simulink library "ZumoBotLib"  (R2014a)
settings: Solver=ode45  StartTime=0.0  StopTime=10.0  RelTol=1e-3
libraries: simulink x4, arduinolib x4
settings Model: Creator=cgupta  LastModifiedBy=cgupta

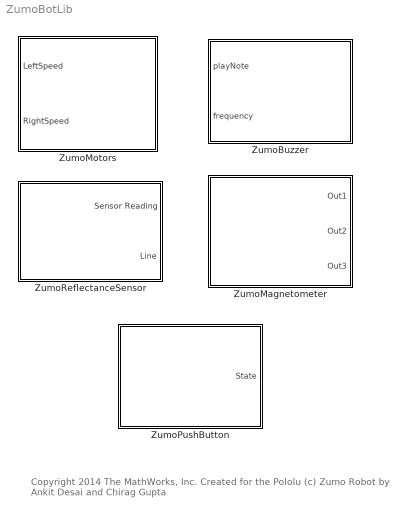
== system ZumoBotLib ==
  note: Copyright 2014 The MathWorks, Inc.
      | Created for the Pololu (c)  Zumo Robot by Ankit Desai and Chirag Gupta
  ZumoBuzzer : Subsystem  mask(Zumo Buzzer){}
      mask help:
      | This block provides access to the piezo buzzer on the ZumoBot.
      | The Block takes 2 inputs:
      | Enable: That enables the Buzzer
      | Frequency: That plays the specified frequency on the buzzer.
      mask Help:
      | This block provides access to the piezo buzzer on the ZumoBot.
      | The Block takes 2 inputs:
      | Enable: That enables the Buzzer
      | Frequency: That plays the specified frequency on the buzzer.
      mask Display:
      | image('zumobuzzer.jpg')
      | port_label('input',1,'Enable')
      | port_label('input',2,'Frequency')
  ZumoMagnetometer : Subsystem  mask(Zumo LSM303 Block){sampletime_lsm=0.2, debug_lsm=off, minX_lsm=-2048, maxX_lsm=2048, minY_lsm=-2048, maxY_lsm=2048, minZ_lsm=-4096, maxZ_lsm=4096}
      mask prompts: sampletime_lsm "Sample Time"; debug_lsm "Debug"; minX_lsm "Min Compass X"; maxX_lsm "Max Compass X"; minY_lsm "Min Compass Y"; maxY_lsm "Max Compass Y"; minZ_lsm "Min Compass Z"; maxZ_lsm "Max Compass Z"
      mask help:
      | This block provides acceleration as well as compass values.
      |
      | The output ports are: Acceleration and Compass respectively.
      |
      | The individual X, Y and Z values can be accessed from the bus for each.
      |
      | The SampleTime Parameter should be greater that 0.01.
      | The Debug checkbox enables debug Serial Print.
      |
      | The Min/Max Compass Readings can be calibrated to get accurate readings from the Magnetometer.
      mask Help:
      | This block provides acceleration as well as compass values.
      | 
      | The output ports are: Acceleration and Compass respectively.
      | 
      | The individual X, Y and Z values can be accessed from the bus for each.
      | 
      | The SampleTime Parameter should be greater that 0.01.
      | The Debug checkbox enables debug Serial Print.
      mask Display:
      | image('LSM_Magnetometer.jpg');
      | port_label('output',1,'Acceleration');
      | port_label('output',2,'Compass');
      | port_label('output',3,'Heading');
  ZumoMotors : Subsystem  mask(Zumo Motors){flipLeft=off, flipRight=off}
      mask prompts: flipLeft "Flip Left Motors"; flipRight "Flip Right Motors"
      mask help:
      | This Block allows you to control the speed and direction of the motors of
      | the ZumoBot.
      |
      | The ZumoMotors block accepts speed in the range of -255 to 255 where the
      | negative sign reverse direction of the motor.
      |
      | Incase one of your motors is configured to the contrary (- denotes forward
      | motion), you can set the flipLeft(/Right) motor flag on the block to
      | correct this.
      mask Display:
      | image('ZumoMotors.jpg')
      | port_label('input',1,'LeftSpeed')
      | port_label('input',2,'RightSpeed')
  ZumoPushButton : Subsystem  mask(Zumo Push Button){sampleTime_push=0.2}
      mask prompts: sampleTime_push "Sample Time"
      mask help:
      | This block provides access to the Push Button on the ZumoBot.
      |
      | The State returned is HIGH when the button is pressed, else LOW.
      mask Help:
      | This block provides access to the Push Button on the ZumoBot.
      | 
      | The State returned is HIGH when the button is pressed, else LOW.
      mask Display:
      | image('Zumo_push.jpg');
      | port_label('output',1,'State');
  ZumoReflectanceSensor : Subsystem  mask(Zumo Reflectance Sensor){sampleTime_dd=0.1, emitterPin_dd=255, debug_dd=off}
      mask prompts: sampleTime_dd "Sample Time"; emitterPin_dd "Emitter Pin"; debug_dd "Debug"
      mask help:
      | This is the driver block to access the Reflectance Sensor on the Zumo bot.
      | This block returns the raw sensor values of the each individual sensor as
      | well as the averaged line indicator.
      |
      | The Line Indicator has a value range from 0 - 5000 where 0 represents that
      | the line is underneath sensor 0 and 5000 represents that the line is under
      | sensor 6.
      | The Raw values of each sensor range from 0 - 2000.
      | The SampleTime Parameter should be greater that 0.01.
      | The Debug Checkbox enables debug Serial Print.
      |
      | The Emitter Pin is diasbled at 255, which signifies that the sensor
      | emitters are always on.
      mask TypeOptions emitterPin_dd: 255 | 1 | 0
      mask Display:
      | image('ZumoReflectanceArray.jpg',[0,0,0.75,1]);
      | port_label('output',1,'RawValues');
      | port_label('output',2,'Line');

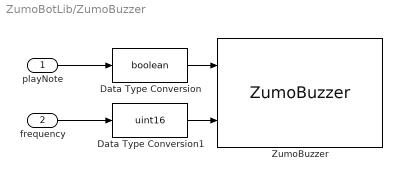
== system ZumoBotLib/ZumoBuzzer ==
  playNote : Inport
  frequency : Inport  Port=2
  Data Type Conversion : DataTypeConversion  OutDataTypeStr=boolean
  Data Type Conversion1 : DataTypeConversion  OutDataTypeStr=uint16
  ZumoBuzzer : S-Function  InitFcn=try, set_param(gcb,'FunctionName','ZumoBuzzer'), end  FunctionName=ZumoBuzzer  SFunctionModules=ZumoBuzzer_wrapper  EnableBusSupport=off  mask(S-Function Builder){frequency_zumobuzzer=0}
      mask prompts: frequency_zumobuzzer "Frequency"
      mask help: Simulink:masks:SFunctionBuilder_MD
      mask init:
      | val = [[.9  0.75 0.75 1 1 .9 .9 1]',[1 1 0.75 0.75 .9 .9 1 .9]'];try , sys = get_param(gcb,'SfunBuilderFcnName');if isempty(sys), sys = get_param(gcb,'FunctionName'); end,catch, sys = get_param(gcb,'FunctionName'); end
      settings: PreSaveFcn=try, set_param(gcb,'FunctionName','ZumoBuzzer'), end  OpenFcn=sfunctionwizard(gcbh)
      mask Display: plot(val(:,1),val(:,2)),disp(sys), port_label('input',1,'playTone'), port_label('input',2,'frequency')
  wires:
  playNote/1 -> Data Type Conversion/1
  Data Type Conversion/1 -> ZumoBuzzer/1
  Data Type Conversion1/1 -> ZumoBuzzer/2
  frequency/1 -> Data Type Conversion1/1

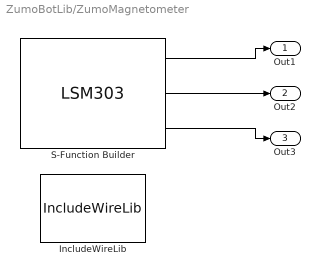
== system ZumoBotLib/ZumoMagnetometer ==
  IncludeWireLib : S-Function  InitFcn=try, set_param(gcb,'FunctionName','IncludeWireLib'), end  FunctionName=IncludeWireLib  SFunctionModules=IncludeWireLib_wrapper  EnableBusSupport=off  mask(S-Function Builder){}
      mask help: Simulink:masks:SFunctionBuilder_MD
      mask init: same as ZumoBotLib/ZumoBuzzer/ZumoBuzzer
      settings: PreSaveFcn=try, set_param(gcb,'FunctionName','IncludeWireLib'), end  OpenFcn=sfunctionwizard(gcbh)
      mask Display:
      | plot(val(:,1),val(:,2))
      | disp(sys)
  S-Function Builder : S-Function  InitFcn=try, set_param(gcb,'FunctionName','LSM303'), end  FunctionName=LSM303  Parameters=sampletime_lsm,boolean(debug_lsm),minX_lsm,maxX_lsm,minY_lsm,maxY_lsm,minZ_lsm,boolean(maxZ_lsm)  SFunctionModules=LSM303_wrapper  EnableBusSupport=off  mask(S-Function Builder){}
      mask help: Simulink:masks:SFunctionBuilder_MD
      mask init: same as ZumoBotLib/ZumoBuzzer/ZumoBuzzer
      settings: PreSaveFcn=try, set_param(gcb,'FunctionName','LSM303'), end  OpenFcn=sfunctionwizard(gcbh)
      mask Display: plot(val(:,1),val(:,2)),disp(sys), port_label('output',1,'Acceleration'), port_label('output',2,'Compass'), port_label('output',3,'Heading')
  Out1 : Outport
  Out2 : Outport  Port=2
  Out3 : Outport  Port=3
  wires:
  S-Function Builder/1 -> Out1/1
  S-Function Builder/2 -> Out2/1
  S-Function Builder/3 -> Out3/1

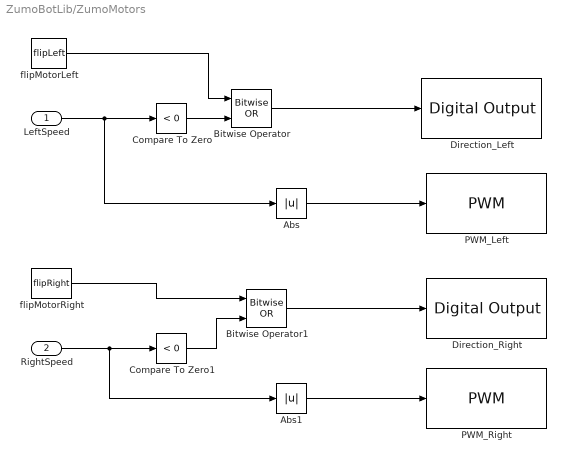
== system ZumoBotLib/ZumoMotors ==
  LeftSpeed : Inport
  RightSpeed : Inport  Port=2
  Abs : Abs  OutDataTypeStr=uint8  SaturateOnIntegerOverflow=on
  Abs1 : Abs  OutDataTypeStr=uint8  SaturateOnIntegerOverflow=on
  Bitwise Operator : simulink/Logic and Bit Operations/Bitwise Operator  logicop=OR  UseBitMask=off  NumInputPorts=2  BitMask=bin2dec('11011001')  BitMaskRealWorld=Stored Integer
  Bitwise Operator1 : simulink/Logic and Bit Operations/Bitwise Operator  logicop=OR  UseBitMask=off  NumInputPorts=2  BitMask=bin2dec('11011001')  BitMaskRealWorld=Stored Integer
  Compare To Zero : simulink/Logic and Bit Operations/Compare To Zero  relop=<  OutDataTypeStr=boolean
  Compare To Zero1 : simulink/Logic and Bit Operations/Compare To Zero  relop=<  OutDataTypeStr=boolean
  Direction_Left : arduinolib/Digital Output  pinNumber=8
  Direction_Right : arduinolib/Digital Output  pinNumber=7
  PWM_Left : arduinolib/PWM  pinNumber=10
  PWM_Right : arduinolib/PWM  pinNumber=9
  flipMotorLeft : Constant  Value=flipLeft  OutDataTypeStr=boolean
  flipMotorRight : Constant  Value=flipRight  OutDataTypeStr=boolean
  wires:
  Compare To Zero/1 -> Bitwise Operator/2
  Abs/1 -> PWM_Left/1
  Abs1/1 -> PWM_Right/1
  flipMotorLeft/1 -> Bitwise Operator/1
  LeftSpeed/1 -> Abs/1, Compare To Zero/1
  flipMotorRight/1 -> Bitwise Operator1/1
  Bitwise Operator1/1 -> Direction_Right/1
  Compare To Zero1/1 -> Bitwise Operator1/2
  Bitwise Operator/1 -> Direction_Left/1
  RightSpeed/1 -> Abs1/1, Compare To Zero1/1

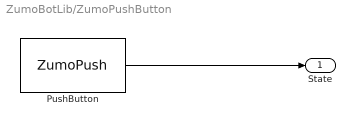
== system ZumoBotLib/ZumoPushButton ==
  PushButton : S-Function  InitFcn=try, set_param(gcb,'FunctionName','ZumoPush'), end  FunctionName=ZumoPush  Parameters=sampleTime_push  SFunctionModules=ZumoPush_wrapper  EnableBusSupport=off  mask(S-Function Builder){}
      mask help: Simulink:masks:SFunctionBuilder_MD
      mask init: same as ZumoBotLib/ZumoBuzzer/ZumoBuzzer
      settings: PreSaveFcn=try, set_param(gcb,'FunctionName','ZumoPush'), end  OpenFcn=sfunctionwizard(gcbh)
      mask Display: plot(val(:,1),val(:,2)),disp(sys), port_label('output',1,'State')
  "State " : Outport
  wires:
  PushButton/1 -> "State "/1

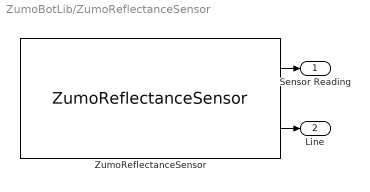
== system ZumoBotLib/ZumoReflectanceSensor ==
  ZumoReflectanceSensor : S-Function  InitFcn=try, set_param(gcb,'FunctionName','ZumoReflectanceSensor'), end  FunctionName=ZumoReflectanceSensor  Parameters=sampleTime_dd,uint8(emitterPin_dd),boolean(debug_dd)  SFunctionModules=ZumoReflectanceSensor_wrapper  EnableBusSupport=off  mask(S-Function Builder){}
      mask help: Simulink:masks:SFunctionBuilder_MD
      mask init: same as ZumoBotLib/ZumoBuzzer/ZumoBuzzer
      settings: PreSaveFcn=try, set_param(gcb,'FunctionName','ZumoReflectanceSensor'), end  OpenFcn=sfunctionwizard(gcbh)
      mask Display: plot(val(:,1),val(:,2)),disp(sys), port_label('output',1,'sensorReading'), port_label('output',2,'line')
  Sensor Reading : Outport
  Line : Outport  Port=2
  wires:
  ZumoReflectanceSensor/2 -> Line/1
  ZumoReflectanceSensor/1 -> Sensor Reading/1
